simulink model "Lab3PartB_2"  (R2021b)
settings: Solver=ode45  StartTime=0.0  StopTime=18  RelTol=1e-3  EnableMultiTasking=on
undefined symbols (not defined in the file or in its folder): DiscIntNeverNeededParam
libraries: simulink x2
settings Model: Creator=Kalai  LastModifiedBy=Gajendra Jayasekera
settings SolverCC: AlgebraicLoopSolver=TrustRegion
settings DataIOCC: LimitDataPoints=on  SaveFormat=Array  ReturnWorkspaceOutputs=off
settings OptimizationCC: LifeSpan=inf
settings DebuggingCC: UnderspecifiedInitializationDetection=Classic  MergeDetectMultiDrivingBlocksExec=none  SolverPrmCheckMsg=warning  SFUnexpectedBacktrackingDiag=warning  SFNoUnconditionalDefaultTransitionDiag=warning  SFExecutionAtInitializationDiag=none  SFMachineParentedDataDiag=warning  ArithmeticOperatorsInVariantConditions=warning
settings HardwareCC: ProdBitPerPointer=32  ProdBitPerSizeT=32  ProdBitPerPtrDiffT=32  ProdLargestAtomicFloat=None  ProdIntDivRoundTo=Undefined  ProdEndianess=Unspecified  ProdWordSize=32  ProdHWDeviceType=32-bit Generic
settings ModelReferenceCC: PropagateSignalLabelsOutOfModel=off
settings SFSimCC: SimUseLocalCustomCode=off  CustomCodeUndefinedFunction=UseInterfaceOnly
settings RTWCC: RTWUseLocalCustomCode=off
settings CodeAppCC: StateflowObjectComments=on
settings GRTTargetCC: TargetLangStandard=C89/C90 (ANSI)
settings ConfigComp: CovMetricSettings=dw  CovSaveCumulativeToWorkspaceVar=on  CovSaveSingleToWorkspaceVar=on  CovExternalEMLEnable=off

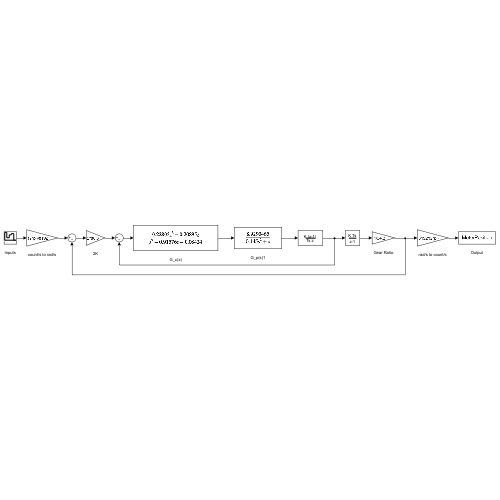
[thumbnail: Simulink's stored preview of the top-level diagram]
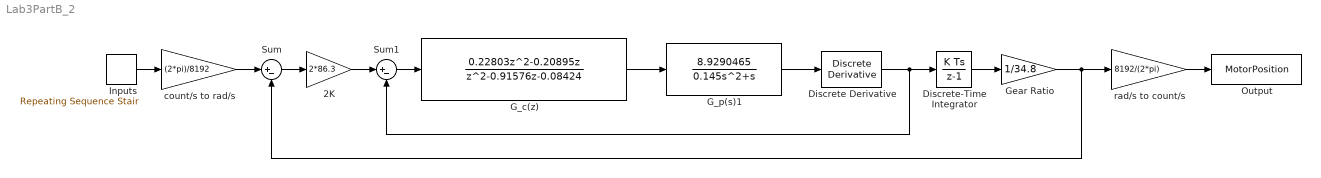
== system Lab3PartB_2 ==
  " 2K" : Gain  Gain=2*86.3
  " G_c(z)" : DiscreteTransferFcn  Numerator=[0.22803 -0.20895 0]  Denominator=[1 -0.91576 -0.08424]  SampleTime=0.009
  " G_p(s)1" : TransferFcn  Numerator=[8.9290465]  Denominator=[0.145 1 0]
  " Gear Ratio" : Gain  Gain=1/34.8
  " Inputs" : simulink/Sources/Repeating Sequence Stair  OutValues=[3072 1024 2048 2560 0].'  tsamp=3.6  OutMin=[]  OutMax=[]  OutDataTypeStr=double  OutputDataTypeScalingMode=double  OutDataType=fixdt(0,8)  ConRadixGroup=Best Precision: Vector-wise  OutScaling=2^-12
  " Output" : ToWorkspace  VariableName=MotorPosition  SaveFormat=Timeseries  SampleTime=-1
  " count/s to rad/s" : Gain  Gain=(2*pi)/8192
  " rad/s to count/s" : Gain  Gain=8192/(2*pi)
  Discrete Derivative : simulink/Discrete/Discrete Derivative  gainval=1.0  ICPrevScaledInput=0.0  OutMin=[]  OutMax=[]  OutDataType=fixdt(1, 16)  OutScaling=2^-10  DoSatur=off
  Discrete-Time Integrator : DiscreteIntegrator  SampleTime=-1  ICPrevOutput=DiscIntNeverNeededParam  ICPrevScaledInput=DiscIntNeverNeededParam
  Sum : Sum  Inputs=|+-
  Sum1 : Sum  Inputs=|+-
  wires:
  " 2K"/1 -> Sum1/1
  " count/s to rad/s"/1 -> Sum/1
  Sum/1 -> " 2K"/1
  " G_p(s)1"/1 -> Discrete Derivative/1
  " rad/s to count/s"/1 -> " Output"/1
  " Gear Ratio"/1 -> " rad/s to count/s"/1, Sum/2
  Discrete-Time Integrator/1 -> " Gear Ratio"/1
  " G_c(z)"/1 -> " G_p(s)1"/1
  Discrete Derivative/1 -> Discrete-Time Integrator/1, Sum1/2
  " Inputs"/1 -> " count/s to rad/s"/1
  Sum1/1 -> " G_c(z)"/1
